simulink model "dlbsTestHarnessBceLoss"  (R2025b)
settings: Solver=VariableStepAuto  StartTime=0.0  StopTime=10.0  RelTol=1e-3
undefined symbols (not defined in the file or in its folder): Y, Y_ref
libraries: dlbsBlockExtractGradientGF x2, dlbsBlockBceLoss x1
settings Model: Creator=lt6037  LastModifiedBy=lt6037

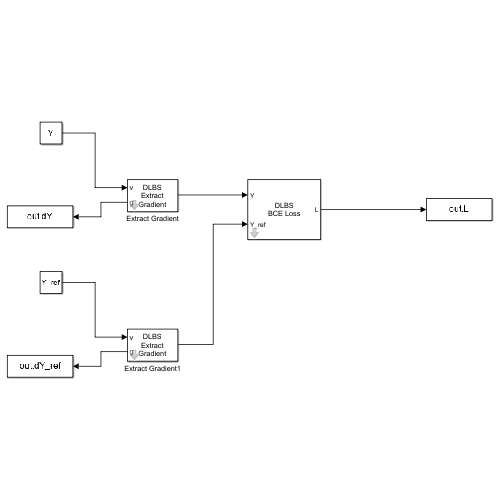
[thumbnail: Simulink's stored preview of the top-level diagram]
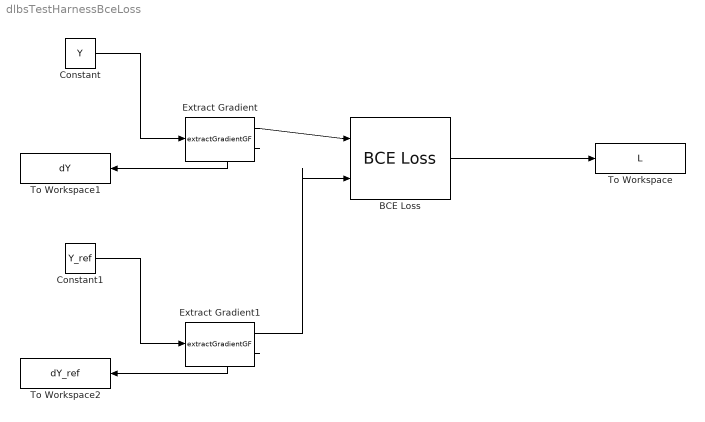
== system dlbsTestHarnessBceLoss ==
  BCE Loss : dlbsBlockBceLoss/BCE Loss
  Constant : Constant  Value=Y  VectorParams1D=off
  Constant1 : Constant  Value=Y_ref  VectorParams1D=off
  Extract Gradient : dlbsBlockExtractGradientGF/extractGradientGF
  Extract Gradient1 : dlbsBlockExtractGradientGF/extractGradientGF
  To Workspace : ToWorkspace  VariableName=L  SaveFormat=Timeseries  SampleTime=-1
      settings: MaxDataPoints=1
  To Workspace1 : ToWorkspace  VariableName=dY  SaveFormat=Timeseries  SampleTime=-1
      settings: MaxDataPoints=1
  To Workspace2 : ToWorkspace  VariableName=dY_ref  SaveFormat=Timeseries  SampleTime=-1
      settings: MaxDataPoints=1
  wires:
  Extract Gradient/2 -> To Workspace1/1
  Constant/1 -> Extract Gradient/1
  BCE Loss/1 -> To Workspace/1
  Constant1/1 -> Extract Gradient1/1
  Extract Gradient1/2 -> To Workspace2/1
  Extract Gradient/1 -> BCE Loss/1
  Extract Gradient1/1 -> BCE Loss/2
